simulink library "liftingBodyTension"  (R2018b)
settings: Solver=VariableStepAuto  StartTime=0.0  StopTime=10.0  RelTol=1e-3
undefined symbols (not defined in the file or in its folder): mag, position
libraries: vectorNormalizer_ul x1
settings Model: Creator=Erin B  LastModifiedBy=Erin B

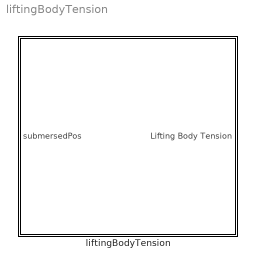
== system liftingBodyTension ==
  liftingBodyTension : Subsystem  mask{pos=position, mag=mag}
      mask prompts: pos "Position of Airborne System"; mag "Magnitude of Tension"

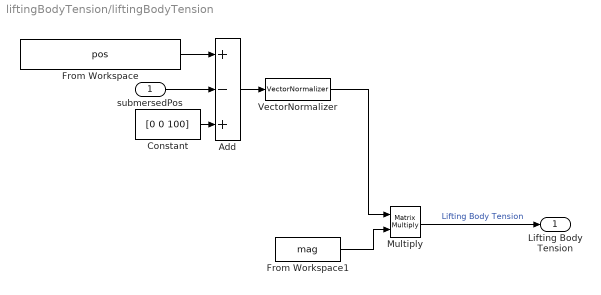
== system liftingBodyTension/liftingBodyTension ==
  submersedPos : Inport
  Add : Sum  Inputs=+-+
  Constant : Constant  Value=[0 0 100]
  From Workspace : FromWorkspace  VariableName=pos  SampleTime=0
  From Workspace1 : FromWorkspace  VariableName=mag  SampleTime=0
  Multiply : Product  Multiplication=Matrix(*)
  "VectorNormalizer " : vectorNormalizer_ul/VectorNormalizer   SystemSampleTime=-1
  Lifting Body Tension : Outport
  wires:
  From Workspace1/1 -> Multiply/2
  "VectorNormalizer "/1 -> Multiply/1
  Multiply/1 -> Lifting Body Tension/1  "Lifting Body Tension"
  From Workspace/1 -> Add/1
  submersedPos/1 -> Add/2
  Add/1 -> "VectorNormalizer "/1
  Constant/1 -> Add/3
